simulink model "amplifier_model"  (R2024a)
settings: Solver=VariableStepAuto  StartTime=0.0  StopTime=20  RelTol=1e-3
settings Model: Creator=alexandr  LastModifiedBy=alexandr

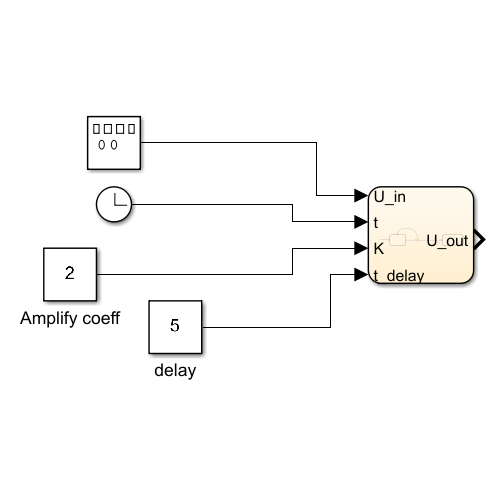
[thumbnail: Simulink's stored preview of the top-level diagram]
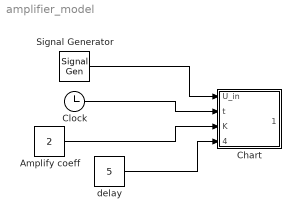
== system amplifier_model ==
  Amplify coeff : Constant  Value=2
  Chart : Stateflow chart  TreatAsAtomicUnit=on
  Clock : Clock
  Signal Generator : SignalGenerator  Units=rad/sec
  delay : Constant  Value=5
  wires:
  Signal Generator/1 -> Chart/1(U_in)
  Clock/1 -> Chart/2(t)
  Amplify coeff/1 -> Chart/3(K)
  delay/1 -> Chart/4(t_delay)

== stateflow chart amplifier_model/Chart ==
  state Delay/
    U_out = 0
  state Amplify/
    U_out = U_in * K
  (junction 11) -> Delay [order 2] : [t < t_delay]
  (default) -> Delay
  Delay -> (junction 11)
  (junction 11) -> Amplify [order 1] : [t >= t_delay]
  data: U_in input; U_out output; t input; K input double =2; t_delay input double =5
